simulink model "VabctoVdq1_1"  (R2021a)
settings: Solver=VariableStepAuto  StartTime=0.0  StopTime=10.0  RelTol=1e-3
settings Model: Creator=danesh  LastModifiedBy=danesh

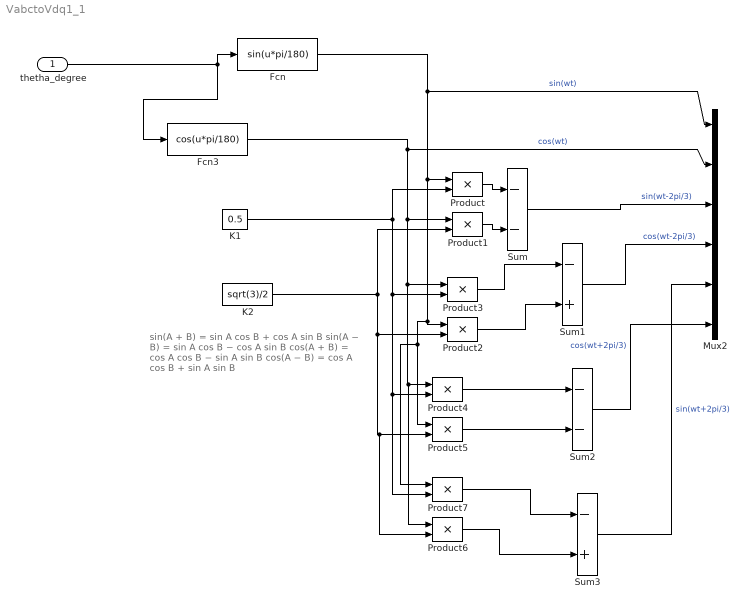
== system VabctoVdq1_1 ==
  note: sin(A + B) = sin A cos B + cos A sin B
      | sin(A − B) = sin A cos B − cos A sin B
      | cos(A + B) = cos A cos B − sin A sin B
      | cos(A − B) = cos A cos B + sin A sin B
  thetha_degree : Inport
  Fcn : Fcn  Expr=sin(u*pi/180)
  Fcn3 : Fcn  Expr=cos(u*pi/180)
  K1 : Constant  Value=0.5
  K2 : Constant  Value=sqrt(3)/2
  Mux2 : Mux  Inputs=6
  Product{,1..7} (8 alike) : Product  InputSameDT=on  SaturateOnIntegerOverflow=on  OutDataTypeStr=Inherit: Same as first input
  Sum : Sum  Inputs=--  InputSameDT=on  SaturateOnIntegerOverflow=on  OutDataTypeStr=Inherit: Same as first input
  Sum1 : Sum  Inputs=-+  InputSameDT=on  SaturateOnIntegerOverflow=on  OutDataTypeStr=Inherit: Same as first input
  Sum2 : Sum  Inputs=--  InputSameDT=on  SaturateOnIntegerOverflow=on  OutDataTypeStr=Inherit: Same as first input
  Sum3 : Sum  Inputs=-+  InputSameDT=on  SaturateOnIntegerOverflow=on  OutDataTypeStr=Inherit: Same as first input
  wires:
  Product2/1 -> Sum1/2
  Sum/1 -> Mux2/3  "sin(wt-2pi/3)"
  Product/1 -> Sum/1
  K2/1 -> Product1/2, Product6/2, Product5/2, Product2/2
  Fcn/1 -> Product/1, Product7/1, Product5/1, Product2/1, Mux2/1  "sin(wt)"
  K1/1 -> Product/2, Product7/2, Product4/2, Product3/2
  Product7/1 -> Sum3/1
  Fcn3/1 -> Product6/1, Product4/1, Product3/1, Product1/1, Mux2/2  "cos(wt)"
  Sum2/1 -> Mux2/6  "cos(wt+2pi/3)"
  thetha_degree/1 -> Fcn3/1, Fcn/1
  Sum3/1 -> Mux2/5  "sin(wt+2pi/3)"
  Product4/1 -> Sum2/1
  Sum1/1 -> Mux2/4  "cos(wt-2pi/3)"
  Product6/1 -> Sum3/2
  Product5/1 -> Sum2/2
  Product3/1 -> Sum1/1
  Product1/1 -> Sum/2
